simulink subsystem "Reefscape_End_Game_sub"  (R2023b)
settings: Solver=VariableStepAuto  StartTime=0.0  StopTime=10.0  RelTol=1e-3
undefined symbols (not defined in the file): Actuator_DC, Actuator_Rev_Startup_Range, Actuator_Rev_Target, Elevator_Height_End_Game, Winch_Hold_DC, Winch_Rev_Target, Winch_Spool_DC
libraries: simulink x4
settings Model: Creator=ander  LastModifiedBy=ander

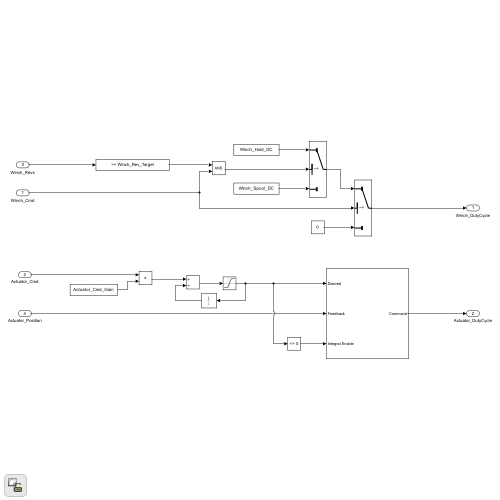
[thumbnail: Simulink's stored preview of the top-level diagram]
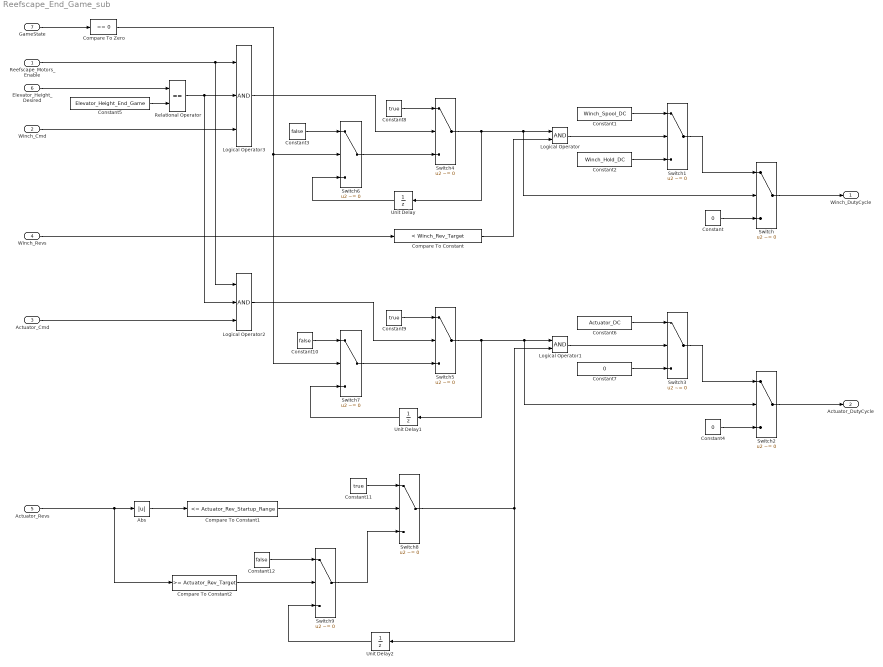
== system Reefscape_End_Game_sub ==
  Reefscape_Motors_Enable : Inport
  Winch_Cmd : Inport  Port=2
  Actuator_Cmd : Inport  Port=3
  Winch_Revs : Inport  Port=4
  Actuator_Revs : Inport  Port=5
  Elevator_Height_Desired : Inport  Port=6
  GameState : Inport  Port=7
  Abs : Abs  SaturateOnIntegerOverflow=off
  Compare To Constant : simulink/Logic and Bit Operations/Compare To Constant  relop=<  const=Winch_Rev_Target  OutDataTypeStr=boolean
  Compare To Constant1 : simulink/Logic and Bit Operations/Compare To Constant  relop=<=  const=Actuator_Rev_Startup_Range  OutDataTypeStr=boolean
  Compare To Constant2 : simulink/Logic and Bit Operations/Compare To Constant  relop=>=  const=Actuator_Rev_Target  OutDataTypeStr=boolean
  Compare To Zero : simulink/Logic and Bit Operations/Compare To Zero  relop===  OutDataTypeStr=boolean
  Constant : Constant  Value=0
  Constant1 : Constant  Value=Winch_Spool_DC
  Constant10 : Constant  Value=false  OutDataTypeStr=boolean
  Constant11 : Constant  Value=true
  Constant12 : Constant  Value=false
  Constant2 : Constant  Value=Winch_Hold_DC
  Constant3 : Constant  Value=false  OutDataTypeStr=boolean
  Constant4 : Constant  Value=0
  Constant5 : Constant  Value=Elevator_Height_End_Game
  Constant6 : Constant  Value=Actuator_DC
  Constant7 : Constant  Value=0
  Constant8 : Constant  Value=true  OutDataTypeStr=boolean
  Constant9 : Constant  Value=true  OutDataTypeStr=boolean
  Logical Operator : Logic  AllPortsSameDT=off  OutDataTypeStr=boolean
  Logical Operator1 : Logic  AllPortsSameDT=off  OutDataTypeStr=boolean
  Logical Operator2 : Logic  Inputs=3  AllPortsSameDT=off  OutDataTypeStr=boolean
  Logical Operator3 : Logic  Inputs=3  AllPortsSameDT=off  OutDataTypeStr=boolean
  Relational Operator : RelationalOperator  Operator===  OutDataTypeStr=boolean  RndMeth=Simplest  InputSameDT=off
  Switch{,1..9} (10 alike) : Switch  Criteria=u2 ~= 0  SaturateOnIntegerOverflow=off  InputSameDT=off
  Unit Delay : UnitDelay  SampleTime=-1  HasFrameUpgradeWarning=on
  Unit Delay1 : UnitDelay  SampleTime=-1  HasFrameUpgradeWarning=on
  Unit Delay2 : UnitDelay  SampleTime=-1  HasFrameUpgradeWarning=on
  Winch_DutyCycle : Outport
  Actuator_DutyCycle : Outport  Port=2
  wires:
  Winch_Revs/1 -> Compare To Constant/1
  Logical Operator/1 -> Switch1/2
  Constant/1 -> Switch/3
  Switch1/1 -> Switch/1
  Switch/1 -> Winch_DutyCycle/1
  Elevator_Height_Desired/1 -> Relational Operator/1
  Constant5/1 -> Relational Operator/2
  Relational Operator/1 -> Logical Operator3/2, Logical Operator2/2
  Switch4/1 -> Switch/2, Logical Operator/1, Unit Delay/1
  Constant8/1 -> Switch4/1
  Constant2/1 -> Switch1/3
  Constant1/1 -> Switch1/1
  Compare To Constant/1 -> Logical Operator/2
  Constant7/1 -> Switch3/3
  Constant9/1 -> Switch5/1
  Switch5/1 -> Switch2/2, Logical Operator1/1, Unit Delay1/1
  Constant6/1 -> Switch3/1
  Switch3/1 -> Switch2/1
  Constant4/1 -> Switch2/3
  Logical Operator1/1 -> Switch3/2
  Switch2/1 -> Actuator_DutyCycle/1
  GameState/1 -> Compare To Zero/1
  Compare To Zero/1 -> Switch6/2, Switch7/2
  Constant3/1 -> Switch6/1
  Winch_Cmd/1 -> Logical Operator3/3
  Unit Delay/1 -> Switch6/3
  Switch6/1 -> Switch4/3
  Logical Operator3/1 -> Switch4/2
  Reefscape_Motors_Enable/1 -> Logical Operator3/1, Logical Operator2/1
  Actuator_Cmd/1 -> Logical Operator2/3
  Logical Operator2/1 -> Switch5/2
  Unit Delay1/1 -> Switch7/3
  Switch7/1 -> Switch5/3
  Constant10/1 -> Switch7/1
  Actuator_Revs/1 -> Abs/1, Compare To Constant2/1
  Switch8/1 -> Unit Delay2/1, Logical Operator1/2
  Compare To Constant1/1 -> Switch8/2
  Unit Delay2/1 -> Switch9/3
  Compare To Constant2/1 -> Switch9/2
  Constant12/1 -> Switch9/1
  Switch9/1 -> Switch8/3
  Constant11/1 -> Switch8/1
  Abs/1 -> Compare To Constant1/1
